simulink model "ShubhamGupta_180749_Lab7_1"  (R2020b)
settings: Solver=ode2  StartTime=0.0  StopTime=100  FixedStep=0.1  RelTol=1e-3
values from neighbouring files (symbols this model uses):
  Kc = x(1)    [ShubhamGupta_180749_Lab7_ISTAE.m]
  Kd = x(7)    [ShubhamGupta_180749_Lab7_ISTAE.m]
  Kp = x(6)    [ShubhamGupta_180749_Lab7_ISTAE.m]
  TD = x(5)    [ShubhamGupta_180749_Lab7_ISTAE.m]
  Td = x(3)    [ShubhamGupta_180749_Lab7_ISTAE.m]
  Theta = x(6)    [ShubhamGupta_180749_Lab7_ISTAE.m]
  Ti = x(2)    [ShubhamGupta_180749_Lab7_ISTAE.m]
  TP = x(4)    [ShubhamGupta_180749_Lab7_ISTAE.m]
settings Model: Creator=Nitin Kaistha  LastModifiedBy=subhamgupta
settings DataIOCC: ReturnWorkspaceOutputs=off

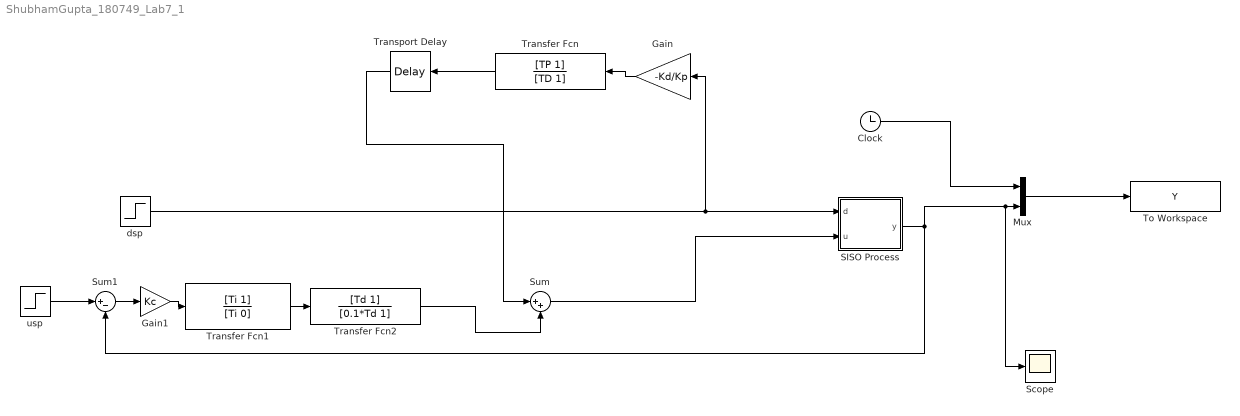
== system ShubhamGupta_180749_Lab7_1 ==
  Clock : Clock
  Gain : Gain  Gain=-Kd/Kp
  Gain1 : Gain  Gain=Kc
  Mux : Mux  Inputs=2
  SISO Process : Subsystem  mask{Kp=1, Tp=1, Kd=1, Td=3}
      mask prompts: Kp "Gp Gain"; Tp "Gp Time Constant"; Kd "Gd Gain"; Td "Gd Time Constant"
  Scope : Scope
  Sum : Sum  Inputs=|++
  Sum1 : Sum  Inputs=|+-
  To Workspace : ToWorkspace  VariableName=Y  SampleTime=-1
  Transfer Fcn : TransferFcn  Numerator=[TP 1]  Denominator=[TD 1]
  Transfer Fcn1 : TransferFcn  Numerator=[Ti 1]  Denominator=[Ti 0]
  Transfer Fcn2 : TransferFcn  Numerator=[Td 1]  Denominator=[0.1*Td 1]
  Transport Delay : TransportDelay  DelayTime=Theta
  dsp : Step  SampleTime=0
  usp : Step  Time=0  After=0  SampleTime=0
  wires:
  dsp/1 -> Gain/1, SISO Process/1(d)
  usp/1 -> Sum1/1
  SISO Process/1(y) -> Scope/1, Mux/2, Sum1/2
  Sum/1 -> SISO Process/2(u)
  Clock/1 -> Mux/1
  Mux/1 -> To Workspace/1
  Gain/1 -> Transfer Fcn/1
  Transfer Fcn/1 -> Transport Delay/1
  Gain1/1 -> Transfer Fcn1/1
  Transfer Fcn1/1 -> Transfer Fcn2/1
  Transfer Fcn2/1 -> Sum/2
  Transport Delay/1 -> Sum/1
  Sum1/1 -> Gain1/1

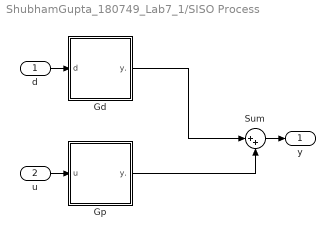
== system ShubhamGupta_180749_Lab7_1/SISO Process ==
  d : Inport
  u : Inport  Port=2
  Gd : Subsystem
  Gp : Subsystem
  Sum : Sum  Inputs=|++
  y : Outport
  wires:
  u/1 -> Gp/1(u)
  Gp/1(y.) -> Sum/2
  Sum/1 -> y/1
  Gd/1(y.) -> Sum/1
  d/1 -> Gd/1(d)

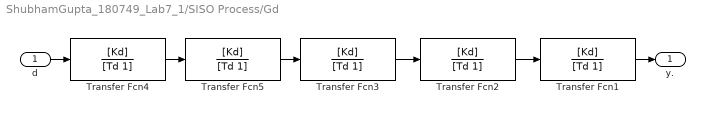
== system ShubhamGupta_180749_Lab7_1/SISO Process/Gd ==
  d : Inport
  Transfer Fcn{1..5} (5 alike) : TransferFcn  Numerator=[Kd]  Denominator=[Td 1]
  y. : Outport
  wires:
  Transfer Fcn4/1 -> Transfer Fcn5/1
  Transfer Fcn5/1 -> Transfer Fcn3/1
  d/1 -> Transfer Fcn4/1
  Transfer Fcn2/1 -> Transfer Fcn1/1
  Transfer Fcn3/1 -> Transfer Fcn2/1
  Transfer Fcn1/1 -> y./1

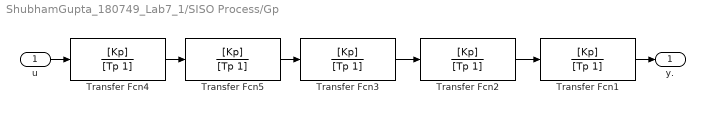
== system ShubhamGupta_180749_Lab7_1/SISO Process/Gp ==
  u : Inport
  Transfer Fcn{1..5} (5 alike) : TransferFcn  Numerator=[Kp]  Denominator=[Tp 1]
  y. : Outport
  wires:
  Transfer Fcn4/1 -> Transfer Fcn5/1
  Transfer Fcn5/1 -> Transfer Fcn3/1
  u/1 -> Transfer Fcn4/1
  Transfer Fcn2/1 -> Transfer Fcn1/1
  Transfer Fcn3/1 -> Transfer Fcn2/1
  Transfer Fcn1/1 -> y./1
